simulink model "odpskok"  (R2020a)
settings: Solver=VariableStepAuto  StartTime=0.0  StopTime=10.0  RelTol=1e-3
values from neighbouring files (symbols this model uses):
  a = 1    [skok.m]    (also in zad2.m)
  b = [1,2,3,4,5,8,11]    [skok.m]    (also in zad2.m = 4)
  c = 50    [skok.m]    (also in zad2.m)
  du = 1    [skok.m]    (also in zad2.m)
  k = 1    [skok.m]    (also in zad2.m)
  u0 = 0    [skok.m]    (also in zad2.m)
  x0 = 0    [skok.m]    (also in zad2.m)
  x10 = 0    [skok.m]    (also in zad2.m)
settings Model: Creator=pc  LastModifiedBy=pc

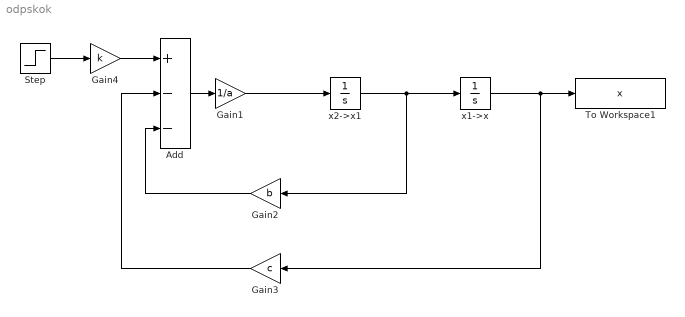
== system odpskok ==
  Add : Sum  Inputs=+--
  Gain1 : Gain  Gain=1/a
  Gain2 : Gain  Gain=b
  Gain3 : Gain  Gain=c
  Gain4 : Gain  Gain=k
  Step : Step  Time=0  Before=u0  After=u0+du  SampleTime=0.01
  To Workspace1 : ToWorkspace  VariableName=x  SampleTime=-1
  x1->x : Integrator  InitialCondition=x0
  x2->x1 : Integrator  InitialCondition=x10
  wires:
  Gain4/1 -> Add/1
  Gain1/1 -> x2->x1/1
  Gain3/1 -> Add/2
  x1->x/1 -> Gain3/1, To Workspace1/1
  Add/1 -> Gain1/1
  Gain2/1 -> Add/3
  Step/1 -> Gain4/1
  x2->x1/1 -> Gain2/1, x1->x/1
